simulink model "SimulinkModel_PID_InitialTest"  (R2020a)
settings: Solver=ode14x  StartTime=0.0  StopTime=SimTime  FixedStep=1/CF  RelTol=1e-3
InitFcn:
  | StartupScript
values from neighbouring files (symbols this model uses):
  Amp_denom = 5    [StartupScript.m]
  Amp_num = 5    [StartupScript.m]
  B = 0.0007    [StartupScript.m]
  CF = 100.0    (= 100)    [StartupScript.m]
  J = 9.545e-6    (= 9.545e-06)    [StartupScript.m]
  K = 11.0    (= 11)    [StartupScript.m]
  Kd = 0.1    [StartupScript.m]
  Ki = 8.9    [StartupScript.m]
  Km = 35.6e-3    (= 0.0356)    [StartupScript.m]
  Kp = 5.9    [StartupScript.m]
  L = 1.320e-3    (= 0.00132)    [StartupScript.m]
  R = 22.8    [StartupScript.m]
  r2d = 180/pi    (= 57.2957795131)    [StartupScript.m]
  sensorGain = 150.0    (= 150)    [StartupScript.m]
settings Model: Creator=nisch  LastModifiedBy=nisch

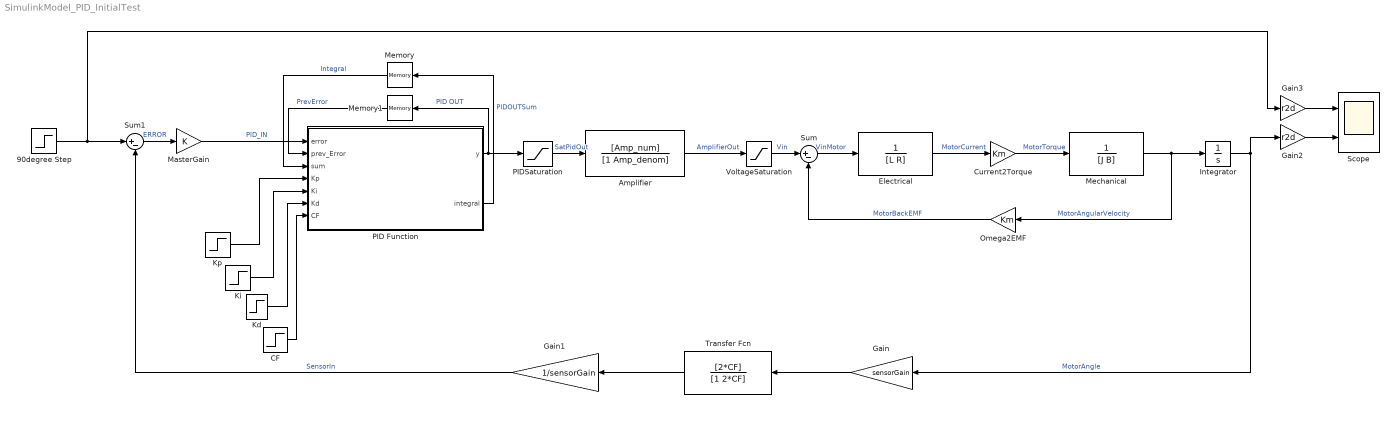
== system SimulinkModel_PID_InitialTest ==
  90degree Step : Step  Time=0  After=pi/2  SampleTime=0
  Amplifier : TransferFcn  Numerator=[Amp_num]  Denominator=[1 Amp_denom]
  CF : Step  Time=0  After=CF  SampleTime=0
  Current2Torque : Gain  Gain=Km
  Electrical : TransferFcn  Denominator=[L R]
  Gain : Gain  Gain=sensorGain
  Gain1 : Gain  Gain=1/sensorGain
  Gain2 : Gain  Gain=r2d
  Gain3 : Gain  Gain=r2d
  Integrator : Integrator
  Kd : Step  Time=0  After=Kd  SampleTime=0
  Ki : Step  Time=0  After=Ki  SampleTime=0
  Kp : Step  Time=0  After=Kp  SampleTime=0
  MasterGain : Gain  Gain=K
  Mechanical : TransferFcn  Denominator=[J B]
  Memory : Memory  InheritSampleTime=on
  Memory1 : Memory  InheritSampleTime=on
  Omega2EMF : Gain  Gain=Km
  PID Function : MATLAB Function  TreatAsAtomicUnit=on
  PIDSaturation : Saturate  UpperLimit=255  LowerLimit=-255
  Scope : Scope  NumInputPorts=2
  Sum : Sum  Inputs=|+-
  Sum1 : Sum  Inputs=|+-
  Transfer Fcn : TransferFcn  Numerator=[2*CF]  Denominator=[1 2*CF]
  VoltageSaturation : Saturate  UpperLimit=24  LowerLimit=-24
  wires:
  Current2Torque/1 -> Mechanical/1  "MotorTorque"
  Electrical/1 -> Current2Torque/1  "MotorCurrent"
  Sum/1 -> Electrical/1  "VinMotor"
  Omega2EMF/1 -> Sum/2  "MotorBackEMF"
  Mechanical/1 -> Integrator/1, Omega2EMF/1  "MotorAngularVelocity"
  PID Function/1(y) -> Memory1/1, PIDSaturation/1  "PID OUT"
  Sum1/1 -> MasterGain/1  "ERROR"
  Integrator/1 -> Gain2/1, Gain/1  "MotorAngle"
  Gain/1 -> Transfer Fcn/1
  Transfer Fcn/1 -> Gain1/1
  Gain1/1 -> Sum1/2  "SensorIn"
  90degree Step/1 -> Gain3/1, Sum1/1
  MasterGain/1 -> PID Function/1(error)  "PID_IN"
  Gain2/1 -> Scope/2
  Gain3/1 -> Scope/1
  CF/1 -> PID Function/7(CF)
  Kd/1 -> PID Function/6(Kd)
  Ki/1 -> PID Function/5(Ki)
  Kp/1 -> PID Function/4(Kp)
  Memory1/1 -> PID Function/2(prev_Error)  "PrevError"
  Memory/1 -> PID Function/3(sum)  "Integral"
  PID Function/2(integral) -> Memory/1  "PIDOUTSum"
  Amplifier/1 -> VoltageSaturation/1  "AmplifierOut"
  VoltageSaturation/1 -> Sum/1  "Vin"
  PIDSaturation/1 -> Amplifier/1  "SatPidOut"

== matlab function SimulinkModel_PID_InitialTest/PID Function ==
  data: error input; y output; prev_Error input; sum input; Kp input; Ki input; Kd input; CF input; integral output
function [y, integral] = fcn(error, prev_Error, sum, Kp, Ki, Kd, CF)

Kp_Term = Kp * error;
Ki_Term = Ki * (sum + error * (1/CF));
Kd_Term = Kd * (error - prev_Error)/(1/CF);

y = Kp_Term + Ki_Term + Kd_Term;
integral = sum + error * (1/CF);
